simulink model "BodyCtrl_RTW"  (Simulink 7.5)
settings: Solver=ode1  SolverMode=SingleTasking  StartTime=0.0  StopTime=inf  FixedStep=0.001  RelTol=1e-3
PreLoadFcn:
  | vehicle = 'Car'; if ~length(which('cmcmd')), cmenv; end
  | BodyCtrl_RTW_bus
  | BodyCtrl_RTW_params
InitFcn:
  | vehicle = 'Car'; if ~length(which('cmcmd')), cmenv; end
  | BodyCtrl_RTW_bus
  | BodyCtrl_RTW_params
undefined symbols (not defined in the file or in its folder): BodyCtrl_k
libraries: CarMaker4SL x1
Description:
  | CarMaker Real-Time Target (generic)
settings Model: Creator=ml  LastModifiedBy=ml  TunableVars=BodyCtrl_k  TunableVarsStorageClass=ExportedGlobal
settings OptimizationCC: InlineParams=on
settings DebuggingCC: SolverPrmCheckMsg=none
settings HardwareCC: TargetHWDeviceType=32-bit Generic  ProdEqTarget=off
settings RTWCC: SystemTargetFile=CarMaker.tlc  TemplateMakefile=CarMaker_unix.tmf  Description=CarMaker Real-Time Target (32-bit)  ProcessScript=CarMaker_make_rtw_hook
settings CodeAppCC: MaxIdLength=63
settings STFCustomTargetCC: ModelReferenceCompliant=off  GeneratePreprocessorConditionals=Disable all  SystemTargetFile=CarMaker.tlc
settings GRTTargetCC: ModelReferenceCompliant=off  ParMdlRefBuildCompliant=off  CompOptLevelCompliant=off  MatFileLogging=off  ExtModeMexFile=noextcomm  RTWCAPISignals=on  RTWCAPIParams=on
settings CustomProperty: DataType=string  Value=..
settings EnumStrPairs: String=Car

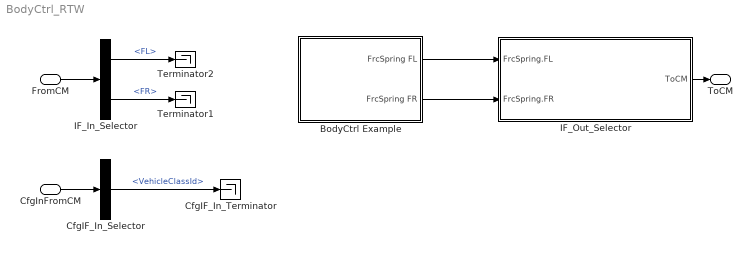
== system BodyCtrl_RTW ==
  FromCM : Inport  UseBusObject=on
      settings: BusObject=cmSuspExtFrcsIn
  CfgInFromCM : Inport  Port=2  UseBusObject=on
      settings: BusObject=cmSuspExtFrcsCfgIn
  BodyCtrl Example : Subsystem
  CfgIF_In_Selector : BusSelector  OutputSignals=VehicleClassId
  CfgIF_In_Terminator : Terminator
  IF_In_Selector : BusSelector  OutputSignals=lSpring.FL,lSpring.FR
  IF_Out_Selector : Subsystem
      settings: OpenFcn=cmSignalSelect('SignalSelection_CB',gcb)
      mask Type: Signal Selection
      mask Description: Signal Selection Block
  Terminator1 : Terminator
  Terminator2 : Terminator
  ToCM : Outport  UseBusObject=on
      settings: BusObject=cmSuspExtFrcsOut
  wires:
  FromCM/1 -> IF_In_Selector/1
  IF_Out_Selector/1(ToCM) -> ToCM/1
  CfgInFromCM/1 -> CfgIF_In_Selector/1
  CfgIF_In_Selector/1 -> CfgIF_In_Terminator/1  "<VehicleClassId>"
  BodyCtrl Example/1(FrcSpring FL) -> IF_Out_Selector/1(FrcSpring.FL)
  BodyCtrl Example/2(FrcSpring FR) -> IF_Out_Selector/2(FrcSpring.FR)
  IF_In_Selector/1 -> Terminator2/1  "<FL>"
  IF_In_Selector/2 -> Terminator1/1  "<FR>"

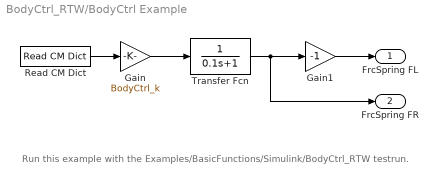
== system BodyCtrl_RTW/BodyCtrl Example ==
  note: Run this example with the Examples/BasicFunctions/Simulink/BodyCtrl_RTW testrun.
  Gain : Gain  Gain=BodyCtrl_k  ParameterDataType=sfix(16)  ParameterScaling=2^0  OutDataType=sfix(16)  OutScaling=2^0  OutDataTypeStr=Inherit: Same as input  ParamDataTypeStr=Inherit: Same as input
  Gain1 : Gain  Gain=-1  ParameterDataType=sfix(16)  ParameterScaling=2^0  OutDataType=sfix(16)  OutScaling=2^0
  Read CM Dict : CarMaker4SL/Read CM Dict  xname=Car.ay  xsync=off
  Transfer Fcn : TransferFcn  Denominator=[0.1 1]
  FrcSpring FL : Outport  OutDataType=sfix(16)  OutScaling=2^0
  FrcSpring FR : Outport  Port=2  OutDataType=sfix(16)  OutScaling=2^0
  wires:
  Transfer Fcn/1 -> FrcSpring FR/1, Gain1/1
  Read CM Dict/1 -> Gain/1
  Gain/1 -> Transfer Fcn/1
  Gain1/1 -> FrcSpring FL/1

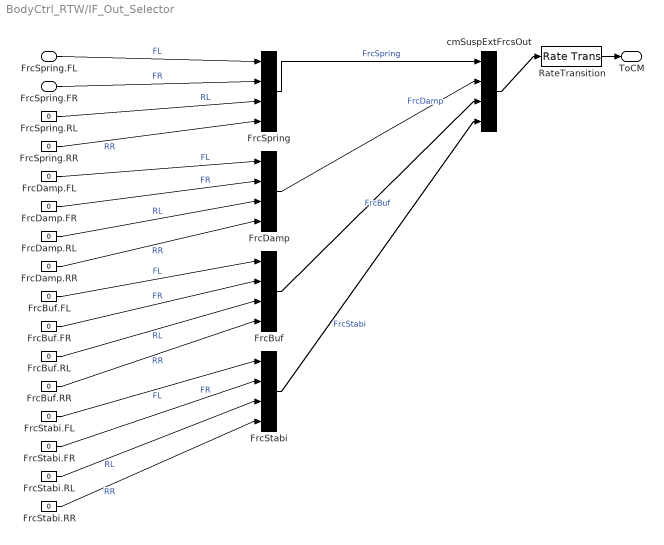
== system BodyCtrl_RTW/IF_Out_Selector ==
  FrcSpring.FL : Inport
  FrcSpring.FR : Inport  Port=2
  FrcBuf : BusCreator
  FrcBuf.FL : Constant  Value=0
  FrcBuf.FR : Constant  Value=0
  FrcBuf.RL : Constant  Value=0
  FrcBuf.RR : Constant  Value=0
  FrcDamp : BusCreator
  FrcDamp.FL : Constant  Value=0
  FrcDamp.FR : Constant  Value=0
  FrcDamp.RL : Constant  Value=0
  FrcDamp.RR : Constant  Value=0
  FrcSpring : BusCreator
  FrcSpring.RL : Constant  Value=0
  FrcSpring.RR : Constant  Value=0
  FrcStabi : BusCreator
  FrcStabi.FL : Constant  Value=0
  FrcStabi.FR : Constant  Value=0
  FrcStabi.RL : Constant  Value=0
  FrcStabi.RR : Constant  Value=0
  RateTransition : RateTransition  OutPortSampleTime=str2num(get_param(bdroot,'FixedStep'))
  cmSuspExtFrcsOut : BusCreator
  ToCM : Outport
  wires:
  RateTransition/1 -> ToCM/1
  cmSuspExtFrcsOut/1 -> RateTransition/1
  FrcSpring/1 -> cmSuspExtFrcsOut/1  "FrcSpring"
  FrcSpring.RL/1 -> FrcSpring/3  "RL"
  FrcSpring.RR/1 -> FrcSpring/4  "RR"
  FrcDamp/1 -> cmSuspExtFrcsOut/2  "FrcDamp"
  FrcDamp.FL/1 -> FrcDamp/1  "FL"
  FrcDamp.FR/1 -> FrcDamp/2  "FR"
  FrcDamp.RL/1 -> FrcDamp/3  "RL"
  FrcDamp.RR/1 -> FrcDamp/4  "RR"
  FrcBuf/1 -> cmSuspExtFrcsOut/3  "FrcBuf"
  FrcBuf.FL/1 -> FrcBuf/1  "FL"
  FrcBuf.FR/1 -> FrcBuf/2  "FR"
  FrcBuf.RL/1 -> FrcBuf/3  "RL"
  FrcBuf.RR/1 -> FrcBuf/4  "RR"
  FrcStabi/1 -> cmSuspExtFrcsOut/4  "FrcStabi"
  FrcStabi.FL/1 -> FrcStabi/1  "FL"
  FrcStabi.FR/1 -> FrcStabi/2  "FR"
  FrcStabi.RL/1 -> FrcStabi/3  "RL"
  FrcStabi.RR/1 -> FrcStabi/4  "RR"
  FrcSpring.FL/1 -> FrcSpring/1  "FL"
  FrcSpring.FR/1 -> FrcSpring/2  "FR"
